simulink model "Laufkatze"  (R2023a)
settings: Solver=FixedStepAuto  StartTime=0.0  StopTime=t  FixedStep=0.001  RelTol=1e-3
InitFcn:
  | % Konstanten
  | m_k = 400; %kg
  | m_l = 200; % kg
  | L_Seil = 10; %m
  | L_Bahn = 60;
  | g = 9.81;
  | t = 20;
  | % Anfangsbedingungen
  | x_dot_initial= 6; %m/s
  | phi_initial = 30 * pi/ 180; % Rad
libraries: simulink x1
settings Model: Creator=nicos  LastModifiedBy=nicos

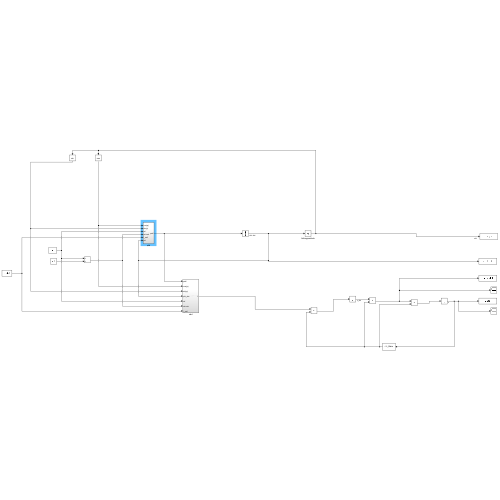
[thumbnail: Simulink's stored preview of the top-level diagram]
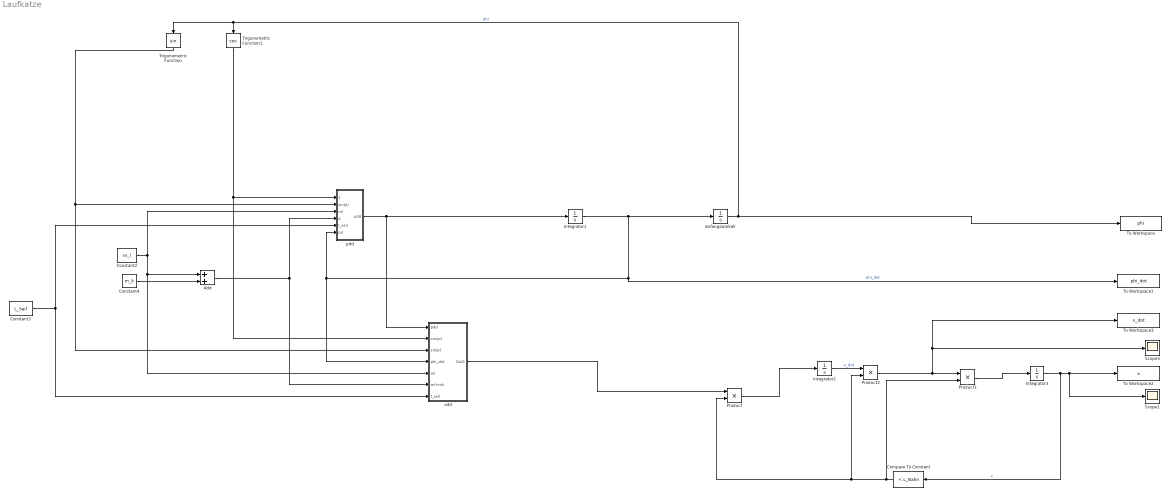
== system Laufkatze ==
  Add : Sum
  Anfangswinkelr : Integrator  InitialCondition=phi_initial
  Compare To Constant : simulink/Logic and Bit Operations/Compare To Constant  relop=<  const=L_Bahn  OutDataTypeStr=boolean
  Constant2 : Constant  Value=m_l
  Constant3 : Constant  Value=L_Seil
  Constant4 : Constant  Value=m_k
  Integrator1 : Integrator
  Integrator2 : Integrator  InitialCondition=x_dot_initial
  Integrator3 : Integrator  UpperSaturationLimit=L_Bahn
  Product : Product
  Product1 : Product
  Product2 : Product
  Scope1 : Scope
  Scope3 : Scope
  To Workspace : ToWorkspace  VariableName=phi  SaveFormat=Timeseries  SampleTime=-1
  To Workspace1 : ToWorkspace  VariableName=phi_dot  SaveFormat=Timeseries  SampleTime=-1
  To Workspace2 : ToWorkspace  VariableName=x  SaveFormat=Timeseries  SampleTime=-1
  To Workspace3 : ToWorkspace  VariableName=x_dot  SaveFormat=Timeseries  SampleTime=-1
  Trigonometric Function : Trigonometry
  Trigonometric Function1 : Trigonometry  Operator=cos
  pdd : Subsystem
  xdd : Subsystem
  wires:
  Anfangswinkelr/1 -> To Workspace/1, Trigonometric Function/1, Trigonometric Function1/1  "phi"
  Integrator1/1 -> To Workspace1/1, xdd/4(phi_dot), pdd/6(pd), Anfangswinkelr/1  "phi_dot"
  Integrator3/1 -> Compare To Constant/1, Scope1/1, To Workspace2/1  "x"
  Integrator2/1 -> Product2/1  "x_dot"
  Product2/1 -> Product1/1, To Workspace3/1, Scope3/1
  Compare To Constant/1 -> Product1/2, Product/2, Product2/2
  Constant2/1 -> xdd/5(ml), Add/1, pdd/3(ml)
  Constant4/1 -> Add/2
  Trigonometric Function/1 -> xdd/3(sin(p)), pdd/2(sin(p))
  Trigonometric Function1/1 -> xdd/2(cos(p)), pdd/1(cos(p))
  Constant3/1 -> xdd/7(I_seil), pdd/5(I_seil)
  Add/1 -> xdd/6(ml+mk), pdd/4(ml+mk)
  pdd/1(pdd) -> xdd/1(pdd), Integrator1/1
  xdd/1(Out1) -> Product/1
  Product/1 -> Integrator2/1
  Product1/1 -> Integrator3/1

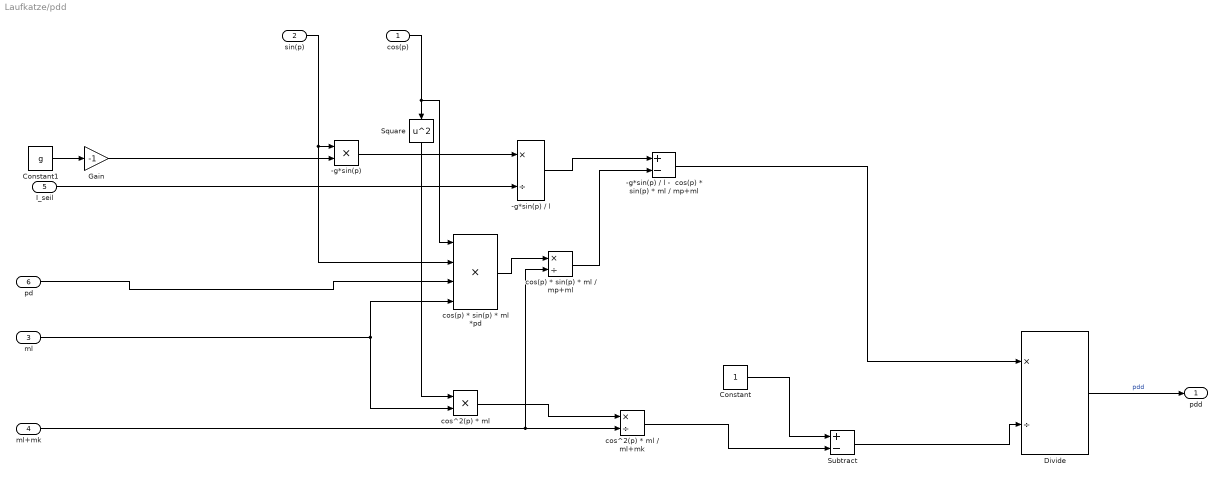
== system Laufkatze/pdd ==
  cos(p) : Inport
  sin(p) : Inport  Port=2
  ml : Inport  Port=3
  ml+mk : Inport  Port=4
  I_seil : Inport  Port=5
  pd : Inport  Port=6
  -g*sin(p) : Product
  -g*sin(p) / l : Product  Inputs=*/
  -g*sin(p) / l -  cos(p) * sin(p) * ml / mp+ml : Sum  Inputs=+-
  Constant : Constant
  Constant1 : Constant  Value=g
  Divide : Product  Inputs=*/
  Gain : Gain  Gain=-1
  Square : Math  Operator=square
  Subtract : Sum  Inputs=+-
  cos(p) * sin(p) * ml *pd : Product  Inputs=4
  cos(p) * sin(p) * ml / mp+ml : Product  Inputs=*/
  cos^2(p) * ml : Product
  cos^2(p) * ml / ml+mk : Product  Inputs=*/
  pdd : Outport
  wires:
  cos(p) * sin(p) * ml / mp+ml/1 -> -g*sin(p) / l -  cos(p) * sin(p) * ml / mp+ml/2
  ml/1 -> cos^2(p) * ml/2, cos(p) * sin(p) * ml *pd/4
  Constant1/1 -> Gain/1
  Square/1 -> cos^2(p) * ml/1
  cos(p) * sin(p) * ml *pd/1 -> cos(p) * sin(p) * ml / mp+ml/1
  ml+mk/1 -> cos(p) * sin(p) * ml / mp+ml/2, cos^2(p) * ml / ml+mk/2
  cos(p)/1 -> cos(p) * sin(p) * ml *pd/1, Square/1
  cos^2(p) * ml / ml+mk/1 -> Subtract/2
  -g*sin(p) / l/1 -> -g*sin(p) / l -  cos(p) * sin(p) * ml / mp+ml/1
  cos^2(p) * ml/1 -> cos^2(p) * ml / ml+mk/1
  Constant/1 -> Subtract/1
  -g*sin(p) / l -  cos(p) * sin(p) * ml / mp+ml/1 -> Divide/1
  -g*sin(p)/1 -> -g*sin(p) / l/1
  sin(p)/1 -> cos(p) * sin(p) * ml *pd/2, -g*sin(p)/1
  Subtract/1 -> Divide/2
  Gain/1 -> -g*sin(p)/2
  Divide/1 -> pdd/1  "pdd"
  I_seil/1 -> -g*sin(p) / l/2
  pd/1 -> cos(p) * sin(p) * ml *pd/3

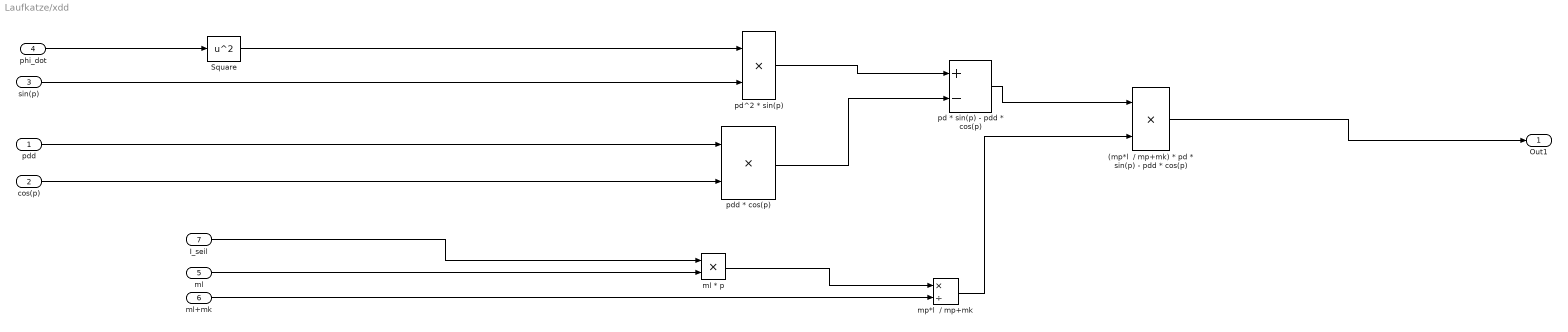
== system Laufkatze/xdd ==
  pdd : Inport
  cos(p) : Inport  Port=2
  sin(p) : Inport  Port=3
  phi_dot : Inport  Port=4
  ml : Inport  Port=5
  ml+mk : Inport  Port=6
  I_seil : Inport  Port=7
  "(mp*l  / mp+mk) * pd * sin(p) - pdd * cos(p) " : Product
  Square : Math  Operator=square
  ml * p : Product
  mp*l  / mp+mk : Product  Inputs=*/
  "pd * sin(p) - pdd * cos(p) " : Sum  Inputs=+-
  pd^2 * sin(p) : Product
  pdd * cos(p) : Product
  Out1 : Outport
  wires:
  phi_dot/1 -> Square/1
  ml * p/1 -> mp*l  / mp+mk/1
  Square/1 -> pd^2 * sin(p)/1
  ml/1 -> ml * p/2
  pdd * cos(p)/1 -> "pd * sin(p) - pdd * cos(p) "/2
  pd^2 * sin(p)/1 -> "pd * sin(p) - pdd * cos(p) "/1
  "pd * sin(p) - pdd * cos(p) "/1 -> "(mp*l  / mp+mk) * pd * sin(p) - pdd * cos(p) "/1
  sin(p)/1 -> pd^2 * sin(p)/2
  cos(p)/1 -> pdd * cos(p)/2
  I_seil/1 -> ml * p/1
  "(mp*l  / mp+mk) * pd * sin(p) - pdd * cos(p) "/1 -> Out1/1
  pdd/1 -> pdd * cos(p)/1
  ml+mk/1 -> mp*l  / mp+mk/2
  mp*l  / mp+mk/1 -> "(mp*l  / mp+mk) * pd * sin(p) - pdd * cos(p) "/2
